simulink model "FormalArchitecture"  (R2022a)
settings: Solver=VariableStepAuto  StartTime=0.0  StopTime=10.0  RelTol=1e-3
settings Model: Creator=jdelolmo  LastModifiedBy=jdelolmo

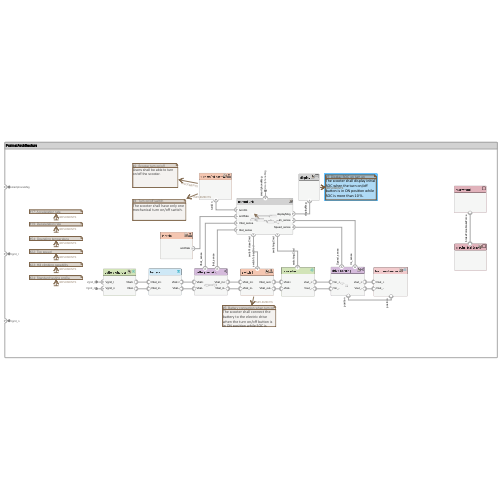
[thumbnail: Simulink's stored preview of the top-level diagram]
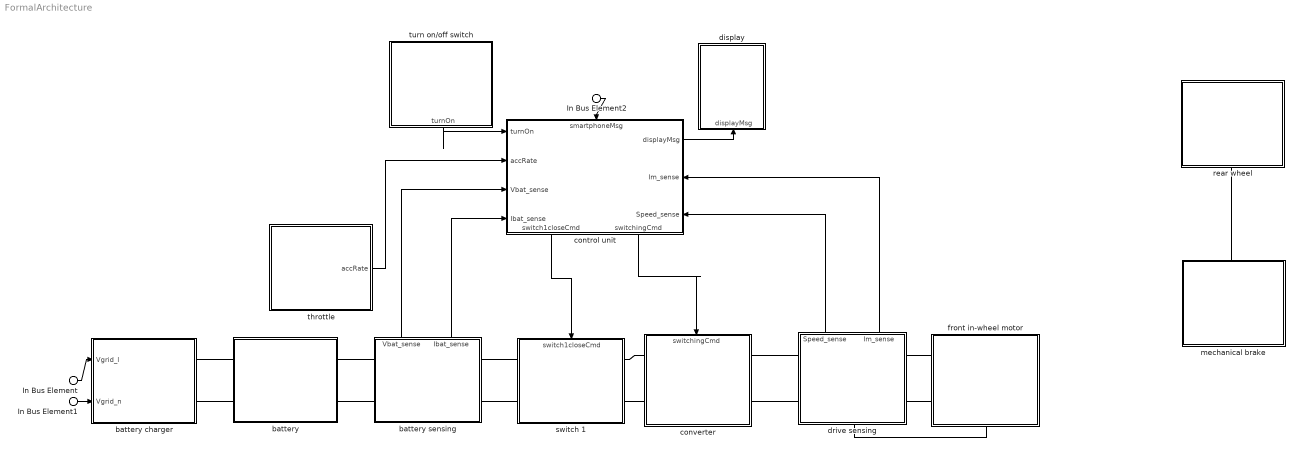
== system FormalArchitecture ==
  In Bus Element2 : Inport  PortName=smartphoneMsg
  In Bus Element : Inport  Port=2  PortName=Vgrid_l
  In Bus Element1 : Inport  Port=3  PortName=Vgrid_n
  battery : Subsystem
      settings: PortSchema="{\"entries\":[{\"content\":{\"headerSize\":26,\"margin\":15,\"minimumSpacing\":25,\"sides\":[{\"content\":{\"connectorIds\":[\"RConn1\",\"RConn2\"]},\"type\":\"ConnectorPlacement.EquallySpacedRectSide\",\"uuid\":\"ee500202-9322-4fb0-a7cb-dad4ec0e2ec3\"},{\"content\":{\"connectorIds\":[\"RConn3\",\"RConn4\"],\"side\":\"RIGHT\"},\"type\":\"ConnectorPlacement.EquallySpacedRectSide\",\"uuid\":\"837fb5dd-499e-46ad-8a25-662d532e1a52\"},{\"content\":{\"connectorIds\":[],\"side\":\"TOP\"},\"type\":\"ConnectorPlacement.EquallySpacedRectSide\",\"uuid\":\"1d32fa59-c030-426a-a0dc-2698c9a02a9b\"},{\"content\":{\"connectorIds\":[],\"side\":\"BOTTOM\"},\"type\":\"ConnectorPlacement.EquallySpacedRectSide\",\"uuid\":\"eb3de403-861e-4d45-8877-523b8cecc4fc\"}]},\"type\":\"ConnectorPlacement.EquallySpacedConnector\",\"uuid\":\"b24d61c9-c26d-4c33-81cf-af7207f0b73c\"}],\"packageUris\":[\"http://schema.mathworks.com/mf0/Connector/R2020b\"],\"version\":\"1.0\"}"
  battery charger : Subsystem
      settings: PortSchema="{\"entries\":[{\"content\":{\"headerSize\":26,\"margin\":15,\"minimumSpacing\":25,\"sides\":[{\"content\":{\"connectorIds\":[\"In1\",\"In2\"]},\"type\":\"ConnectorPlacement.EquallySpacedRectSide\",\"uuid\":\"77baa894-24de-420f-bb05-d29ca1eca7c3\"},{\"content\":{\"connectorIds\":[\"RConn1\",\"RConn2\"],\"side\":\"RIGHT\"},\"type\":\"ConnectorPlacement.EquallySpacedRectSide\",\"uuid\":\"fcd1216d-879c-477b-b249-00119a9fcd22\"},{\"content\":{\"connectorIds\":[],\"side\":\"TOP\"},\"type\":\"ConnectorPlacement.EquallySpacedRectSide\",\"uuid\":\"8485fad0-b9d7-4909-af21-eb521f98cd52\"}]},\"type\":\"ConnectorPlacement.EquallySpacedConnector\",\"uuid\":\"ff53bada-a376-4b82-92cc-106e9afccafe\"}],\"packageUris\":[\"http://schema.mathworks.com/mf0/Connector/R2020b\"],\"version\":\"1.0\"}"
  battery sensing : Subsystem
      settings: PortSchema="{\"entries\":[{\"content\":{\"headerSize\":26,\"margin\":15,\"minimumSpacing\":25,\"sides\":[{\"content\":{\"connectorIds\":[\"LConn1\",\"LConn2\"]},\"type\":\"ConnectorPlacement.EquallySpacedRectSide\",\"uuid\":\"77baa894-24de-420f-bb05-d29ca1eca7c3\"},{\"content\":{\"connectorIds\":[\"RConn1\",\"RConn2\"],\"side\":\"RIGHT\"},\"type\":\"ConnectorPlacement.EquallySpacedRectSide\",\"uuid\":\"fcd1216d-879c-477b-b249-00119a9fcd22\"},{\"content\":{\"connectorIds\":[\"Out2\",\"Out1\"],\"side\":\"TOP\"},\"type\":\"ConnectorPlacement.EquallySpacedRectSide\",\"uuid\":\"8485fad0-b9d7-4909-af21-eb521f98cd52\"},{\"content\":{\"connectorIds\":[],\"side\":\"BOTTOM\"},\"type\":\"ConnectorPlacement.EquallySpacedRectSide\",\"uuid\":\"41cb2969-f54e-4140-878a-5f5a3199a51a\"}]},\"type\":\"ConnectorPlacement.EquallySpacedConnector\",\"uuid\":\"ff53bada-a376-4b82-92cc-106e9afccafe\"}],\"packageUris\":[\"http://schema.mathworks.com/mf0/Connector/R2020b\"],\"version\":\"1.0\"}"
  control unit : Subsystem
      settings: PortSchema="{\"entries\":[{\"content\":{\"headerSize\":26,\"margin\":15,\"minimumSpacing\":25,\"sides\":[{\"content\":{\"connectorIds\":[\"In6\",\"In7\",\"In4\",\"In5\"]},\"type\":\"ConnectorPlacement.EquallySpacedRectSide\",\"uuid\":\"77baa894-24de-420f-bb05-d29ca1eca7c3\"},{\"content\":{\"connectorIds\":[\"Out1\",\"In2\",\"In3\"],\"side\":\"RIGHT\"},\"type\":\"ConnectorPlacement.EquallySpacedRectSide\",\"uuid\":\"fcd1216d-879c-477b-b249-00119a9fcd22\"},{\"content\":{\"connectorIds\":[\"In1\"],\"side\":\"TOP\"},\"type\":\"ConnectorPlacement.EquallySpacedRectSide\",\"uuid\":\"8485fad0-b9d7-4909-af21-eb521f98cd52\"},{\"content\":{\"connectorIds\":[\"Out3\",\"Out2\"],\"side\":\"BOTTOM\"},\"type\":\"ConnectorPlacement.EquallySpacedRectSide\",\"uuid\":\"7527fd4a-b56c-444b-9faf-560b8cff8cb7\"}]},\"type\":\"ConnectorPlacement.EquallySpacedConnector\",\"uuid\":\"ff53bada-a376-4b82-92cc-106e9afccafe\"}],\"packageUris\":[\"http://schema.mathworks.com/mf0/Connector/R2020b\"],\"version\":\"1.0\"}"
  converter : Subsystem
      settings: PortSchema="{\"entries\":[{\"content\":{\"headerSize\":26,\"margin\":15,\"minimumSpacing\":25,\"sides\":[{\"content\":{\"connectorIds\":[\"LConn1\",\"LConn2\"]},\"type\":\"ConnectorPlacement.EquallySpacedRectSide\",\"uuid\":\"77baa894-24de-420f-bb05-d29ca1eca7c3\"},{\"content\":{\"connectorIds\":[\"RConn1\",\"RConn2\"],\"side\":\"RIGHT\"},\"type\":\"ConnectorPlacement.EquallySpacedRectSide\",\"uuid\":\"fcd1216d-879c-477b-b249-00119a9fcd22\"},{\"content\":{\"connectorIds\":[\"In1\"],\"side\":\"TOP\"},\"type\":\"ConnectorPlacement.EquallySpacedRectSide\",\"uuid\":\"8485fad0-b9d7-4909-af21-eb521f98cd52\"}]},\"type\":\"ConnectorPlacement.EquallySpacedConnector\",\"uuid\":\"ff53bada-a376-4b82-92cc-106e9afccafe\"}],\"packageUris\":[\"http://schema.mathworks.com/mf0/Connector/R2020b\"],\"version\":\"1.0\"}"
  display : Subsystem
      settings: PortSchema="{\"entries\":[{\"content\":{\"headerSize\":26,\"margin\":15,\"minimumSpacing\":25,\"sides\":[{\"content\":{\"connectorIds\":[]},\"type\":\"ConnectorPlacement.EquallySpacedRectSide\",\"uuid\":\"77baa894-24de-420f-bb05-d29ca1eca7c3\"},{\"content\":{\"connectorIds\":[],\"side\":\"RIGHT\"},\"type\":\"ConnectorPlacement.EquallySpacedRectSide\",\"uuid\":\"fcd1216d-879c-477b-b249-00119a9fcd22\"},{\"content\":{\"connectorIds\":[],\"side\":\"TOP\"},\"type\":\"ConnectorPlacement.EquallySpacedRectSide\",\"uuid\":\"8485fad0-b9d7-4909-af21-eb521f98cd52\"},{\"content\":{\"connectorIds\":[\"In1\"],\"side\":\"BOTTOM\"},\"type\":\"ConnectorPlacement.EquallySpacedRectSide\",\"uuid\":\"2af0670b-3d52-4fa1-839f-7a09c90230ed\"}]},\"type\":\"ConnectorPlacement.EquallySpacedConnector\",\"uuid\":\"ff53bada-a376-4b82-92cc-106e9afccafe\"}],\"packageUris\":[\"http://schema.mathworks.com/mf0/Connector/R2020b\"],\"version\":\"1.0\"}"
  drive sensing : Subsystem
      settings: PortSchema="{\"entries\":[{\"content\":{\"headerSize\":26,\"margin\":15,\"minimumSpacing\":25,\"sides\":[{\"content\":{\"connectorIds\":[\"LConn1\",\"LConn2\"]},\"type\":\"ConnectorPlacement.EquallySpacedRectSide\",\"uuid\":\"77baa894-24de-420f-bb05-d29ca1eca7c3\"},{\"content\":{\"connectorIds\":[\"RConn2\",\"RConn3\"],\"side\":\"RIGHT\"},\"type\":\"ConnectorPlacement.EquallySpacedRectSide\",\"uuid\":\"fcd1216d-879c-477b-b249-00119a9fcd22\"},{\"content\":{\"connectorIds\":[\"Out1\",\"Out2\"],\"side\":\"TOP\"},\"type\":\"ConnectorPlacement.EquallySpacedRectSide\",\"uuid\":\"8485fad0-b9d7-4909-af21-eb521f98cd52\"},{\"content\":{\"connectorIds\":[\"RConn1\"],\"side\":\"BOTTOM\"},\"type\":\"ConnectorPlacement.EquallySpacedRectSide\",\"uuid\":\"d4cb5d60-5908-4c53-8bc7-b25c3bd545d1\"}]},\"type\":\"ConnectorPlacement.EquallySpacedConnector\",\"uuid\":\"ff53bada-a376-4b82-92cc-106e9afccafe\"}],\"packageUris\":[\"http://schema.mathworks.com/mf0/Connector/R2020b\"],\"version\":\"1.0\"}"
  front in-wheel motor : Subsystem
      settings: PortSchema="{\"entries\":[{\"content\":{\"headerSize\":26,\"margin\":15,\"minimumSpacing\":25,\"sides\":[{\"content\":{\"connectorIds\":[\"LConn1\",\"LConn2\"]},\"type\":\"ConnectorPlacement.EquallySpacedRectSide\",\"uuid\":\"77baa894-24de-420f-bb05-d29ca1eca7c3\"},{\"content\":{\"connectorIds\":[],\"side\":\"RIGHT\"},\"type\":\"ConnectorPlacement.EquallySpacedRectSide\",\"uuid\":\"fcd1216d-879c-477b-b249-00119a9fcd22\"},{\"content\":{\"connectorIds\":[],\"side\":\"TOP\"},\"type\":\"ConnectorPlacement.EquallySpacedRectSide\",\"uuid\":\"8485fad0-b9d7-4909-af21-eb521f98cd52\"},{\"content\":{\"connectorIds\":[\"RConn1\"],\"side\":\"BOTTOM\"},\"type\":\"ConnectorPlacement.EquallySpacedRectSide\",\"uuid\":\"b1cf9e87-5a5a-4f73-9ce1-9d94c90c7687\"}]},\"type\":\"ConnectorPlacement.EquallySpacedConnector\",\"uuid\":\"ff53bada-a376-4b82-92cc-106e9afccafe\"}],\"packageUris\":[\"http://schema.mathworks.com/mf0/Connector/R2020b\"],\"version\":\"1.0\"}"
  mechanical brake : Subsystem
      settings: PortSchema="{\"entries\":[{\"content\":{\"headerSize\":26,\"margin\":15,\"minimumSpacing\":25,\"sides\":[{\"content\":{\"connectorIds\":[]},\"type\":\"ConnectorPlacement.EquallySpacedRectSide\",\"uuid\":\"77baa894-24de-420f-bb05-d29ca1eca7c3\"},{\"content\":{\"connectorIds\":[],\"side\":\"RIGHT\"},\"type\":\"ConnectorPlacement.EquallySpacedRectSide\",\"uuid\":\"fcd1216d-879c-477b-b249-00119a9fcd22\"},{\"content\":{\"connectorIds\":[\"LConn1\"],\"side\":\"TOP\"},\"type\":\"ConnectorPlacement.EquallySpacedRectSide\",\"uuid\":\"8485fad0-b9d7-4909-af21-eb521f98cd52\"}]},\"type\":\"ConnectorPlacement.EquallySpacedConnector\",\"uuid\":\"ff53bada-a376-4b82-92cc-106e9afccafe\"}],\"packageUris\":[\"http://schema.mathworks.com/mf0/Connector/R2020b\"],\"version\":\"1.0\"}"
  rear wheel : Subsystem
      settings: PortSchema="{\"entries\":[{\"content\":{\"headerSize\":26,\"margin\":15,\"minimumSpacing\":25,\"sides\":[{\"content\":{\"connectorIds\":[]},\"type\":\"ConnectorPlacement.EquallySpacedRectSide\",\"uuid\":\"77baa894-24de-420f-bb05-d29ca1eca7c3\"},{\"content\":{\"connectorIds\":[],\"side\":\"RIGHT\"},\"type\":\"ConnectorPlacement.EquallySpacedRectSide\",\"uuid\":\"fcd1216d-879c-477b-b249-00119a9fcd22\"},{\"content\":{\"connectorIds\":[],\"side\":\"TOP\"},\"type\":\"ConnectorPlacement.EquallySpacedRectSide\",\"uuid\":\"8485fad0-b9d7-4909-af21-eb521f98cd52\"},{\"content\":{\"connectorIds\":[\"RConn1\"],\"side\":\"BOTTOM\"},\"type\":\"ConnectorPlacement.EquallySpacedRectSide\",\"uuid\":\"21d572fb-02a4-48d3-884f-e95f709af539\"}]},\"type\":\"ConnectorPlacement.EquallySpacedConnector\",\"uuid\":\"ff53bada-a376-4b82-92cc-106e9afccafe\"}],\"packageUris\":[\"http://schema.mathworks.com/mf0/Connector/R2020b\"],\"version\":\"1.0\"}"
  switch 1 : Subsystem
      settings: PortSchema="{\"entries\":[{\"content\":{\"headerSize\":26,\"margin\":15,\"minimumSpacing\":25,\"sides\":[{\"content\":{\"connectorIds\":[\"LConn1\",\"LConn2\"]},\"type\":\"ConnectorPlacement.EquallySpacedRectSide\",\"uuid\":\"77baa894-24de-420f-bb05-d29ca1eca7c3\"},{\"content\":{\"connectorIds\":[\"RConn1\",\"RConn2\"],\"side\":\"RIGHT\"},\"type\":\"ConnectorPlacement.EquallySpacedRectSide\",\"uuid\":\"fcd1216d-879c-477b-b249-00119a9fcd22\"},{\"content\":{\"connectorIds\":[\"In1\"],\"side\":\"TOP\"},\"type\":\"ConnectorPlacement.EquallySpacedRectSide\",\"uuid\":\"8485fad0-b9d7-4909-af21-eb521f98cd52\"}]},\"type\":\"ConnectorPlacement.EquallySpacedConnector\",\"uuid\":\"ff53bada-a376-4b82-92cc-106e9afccafe\"}],\"packageUris\":[\"http://schema.mathworks.com/mf0/Connector/R2020b\"],\"version\":\"1.0\"}"
  throttle : Subsystem
      settings: PortSchema="{\"entries\":[{\"content\":{\"headerSize\":26,\"margin\":15,\"minimumSpacing\":25,\"sides\":[{\"content\":{\"connectorIds\":[]},\"type\":\"ConnectorPlacement.EquallySpacedRectSide\",\"uuid\":\"77baa894-24de-420f-bb05-d29ca1eca7c3\"},{\"content\":{\"connectorIds\":[\"Out1\"],\"side\":\"RIGHT\"},\"type\":\"ConnectorPlacement.EquallySpacedRectSide\",\"uuid\":\"fcd1216d-879c-477b-b249-00119a9fcd22\"},{\"content\":{\"connectorIds\":[],\"side\":\"TOP\"},\"type\":\"ConnectorPlacement.EquallySpacedRectSide\",\"uuid\":\"8485fad0-b9d7-4909-af21-eb521f98cd52\"}]},\"type\":\"ConnectorPlacement.EquallySpacedConnector\",\"uuid\":\"ff53bada-a376-4b82-92cc-106e9afccafe\"}],\"packageUris\":[\"http://schema.mathworks.com/mf0/Connector/R2020b\"],\"version\":\"1.0\"}"
  turn on/off switch : Subsystem
      settings: PortSchema="{\"entries\":[{\"content\":{\"headerSize\":26,\"margin\":15,\"minimumSpacing\":25,\"sides\":[{\"content\":{\"connectorIds\":[]},\"type\":\"ConnectorPlacement.EquallySpacedRectSide\",\"uuid\":\"77baa894-24de-420f-bb05-d29ca1eca7c3\"},{\"content\":{\"connectorIds\":[],\"side\":\"RIGHT\"},\"type\":\"ConnectorPlacement.EquallySpacedRectSide\",\"uuid\":\"fcd1216d-879c-477b-b249-00119a9fcd22\"},{\"content\":{\"connectorIds\":[],\"side\":\"TOP\"},\"type\":\"ConnectorPlacement.EquallySpacedRectSide\",\"uuid\":\"8485fad0-b9d7-4909-af21-eb521f98cd52\"},{\"content\":{\"connectorIds\":[\"Out1\"],\"side\":\"BOTTOM\"},\"type\":\"ConnectorPlacement.EquallySpacedRectSide\",\"uuid\":\"39085245-15cc-4ad1-9a37-6dd6a1d598c8\"}]},\"type\":\"ConnectorPlacement.EquallySpacedConnector\",\"uuid\":\"ff53bada-a376-4b82-92cc-106e9afccafe\"}],\"packageUris\":[\"http://schema.mathworks.com/mf0/Connector/R2020b\"],\"version\":\"1.0\"}"
  wires:
  turn on/off switch/1(turnOn) -> control unit/6(turnOn)
  control unit/3(switch1closeCmd) -> switch 1/1(switch1closeCmd)
  control unit/1(displayMsg) -> display/1(displayMsg)
  throttle/1(accRate) -> control unit/7(accRate)
  battery sensing/2(Vbat_sense) -> control unit/4(Vbat_sense)
  battery sensing/1(Ibat_sense) -> control unit/5(Ibat_sense)
  drive sensing/2(Im_sense) -> control unit/2(Im_sense)
  drive sensing/1(Speed_sense) -> control unit/3(Speed_sense)
  In Bus Element/1 -> battery charger/1(Vgrid_l)
  In Bus Element1/1 -> battery charger/2(Vgrid_n)
  In Bus Element2/1 -> control unit/1(smartphoneMsg)
  control unit/2(switchingCmd) -> converter/1(switchingCmd)
  connections:
  converter/LConn1 -- switch 1/RConn1
  converter/LConn2 -- switch 1/RConn2
  switch 1/LConn1 -- battery sensing/RConn1
  switch 1/LConn2 -- battery sensing/RConn2
  converter/RConn1 -- drive sensing/LConn1
  converter/RConn2 -- drive sensing/LConn2
  front in-wheel motor/LConn1 -- drive sensing/RConn2
  front in-wheel motor/LConn2 -- drive sensing/RConn3
  drive sensing/RConn1 -- front in-wheel motor/RConn1
  mechanical brake/LConn1 -- rear wheel/RConn1
  battery sensing/LConn1 -- battery/RConn3
  battery sensing/LConn2 -- battery/RConn4
  battery charger/RConn1 -- battery/RConn1
  battery charger/RConn2 -- battery/RConn2

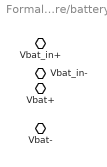
== system FormalArchitecture/battery ==
  Vbat_in+ : PMIOPort  Side=Right
  Vbat_in- : PMIOPort  Port=2  Side=Right
  Vbat+ : PMIOPort  Port=3  Side=Right
  Vbat- : PMIOPort  Port=4  Side=Right

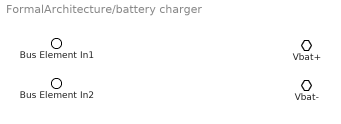
== system FormalArchitecture/battery charger ==
  Bus Element In1 : Inport  PortName=Vgrid_l
  Bus Element In2 : Inport  Port=2  PortName=Vgrid_n
  Vbat+ : PMIOPort  Side=Right
  Vbat- : PMIOPort  Port=2  Side=Right

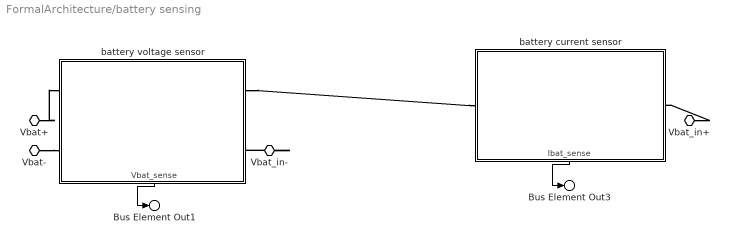
== system FormalArchitecture/battery sensing ==
  battery current sensor : Subsystem
      settings: PortSchema="{\"entries\":[{\"content\":{\"headerSize\":26,\"margin\":15,\"minimumSpacing\":25,\"sides\":[{\"content\":{\"connectorIds\":[\"LConn1\"]},\"type\":\"ConnectorPlacement.EquallySpacedRectSide\",\"uuid\":\"77baa894-24de-420f-bb05-d29ca1eca7c3\"},{\"content\":{\"connectorIds\":[\"RConn1\"],\"side\":\"RIGHT\"},\"type\":\"ConnectorPlacement.EquallySpacedRectSide\",\"uuid\":\"fcd1216d-879c-477b-b249-00119a9fcd22\"},{\"content\":{\"connectorIds\":[],\"side\":\"TOP\"},\"type\":\"ConnectorPlacement.EquallySpacedRectSide\",\"uuid\":\"8485fad0-b9d7-4909-af21-eb521f98cd52\"},{\"content\":{\"connectorIds\":[\"Out1\"],\"side\":\"BOTTOM\"},\"type\":\"ConnectorPlacement.EquallySpacedRectSide\",\"uuid\":\"b087b9fb-29ea-43eb-a167-2ce7aba8e49e\"}]},\"type\":\"ConnectorPlacement.EquallySpacedConnector\",\"uuid\":\"ff53bada-a376-4b82-92cc-106e9afccafe\"}],\"packageUris\":[\"http://schema.mathworks.com/mf0/Connector/R2020b\"],\"version\":\"1.0\"}"
  battery voltage sensor : Subsystem
      settings: PortSchema="{\"entries\":[{\"content\":{\"headerSize\":26,\"margin\":15,\"minimumSpacing\":25,\"sides\":[{\"content\":{\"connectorIds\":[\"LConn1\",\"LConn2\"]},\"type\":\"ConnectorPlacement.EquallySpacedRectSide\",\"uuid\":\"77baa894-24de-420f-bb05-d29ca1eca7c3\"},{\"content\":{\"connectorIds\":[\"RConn1\",\"RConn2\"],\"side\":\"RIGHT\"},\"type\":\"ConnectorPlacement.EquallySpacedRectSide\",\"uuid\":\"fcd1216d-879c-477b-b249-00119a9fcd22\"},{\"content\":{\"connectorIds\":[],\"side\":\"TOP\"},\"type\":\"ConnectorPlacement.EquallySpacedRectSide\",\"uuid\":\"8485fad0-b9d7-4909-af21-eb521f98cd52\"},{\"content\":{\"connectorIds\":[\"Out1\"],\"side\":\"BOTTOM\"},\"type\":\"ConnectorPlacement.EquallySpacedRectSide\",\"uuid\":\"04039fcf-9b1b-4283-ba0c-bcd076f35720\"}]},\"type\":\"ConnectorPlacement.EquallySpacedConnector\",\"uuid\":\"ff53bada-a376-4b82-92cc-106e9afccafe\"}],\"packageUris\":[\"http://schema.mathworks.com/mf0/Connector/R2020b\"],\"version\":\"1.0\"}"
  Vbat+ : PMIOPort  Side=Left
  Vbat- : PMIOPort  Port=2  Side=Left
  Vbat_in+ : PMIOPort  Port=3  Side=Right
  Vbat_in- : PMIOPort  Port=4  Side=Right
  Bus Element Out3 : Outport  PortName=Ibat_sense
  Bus Element Out1 : Outport  Port=2  PortName=Vbat_sense
  wires:
  battery voltage sensor/1(Vbat_sense) -> Bus Element Out1/1
  battery current sensor/1(Ibat_sense) -> Bus Element Out3/1
  connections:
  Vbat+/RConn1 -- battery voltage sensor/LConn1
  Vbat-/RConn1 -- battery voltage sensor/LConn2
  Vbat_in-/RConn1 -- battery voltage sensor/RConn2
  battery voltage sensor/RConn1 -- battery current sensor/LConn1
  Vbat_in+/RConn1 -- battery current sensor/RConn1

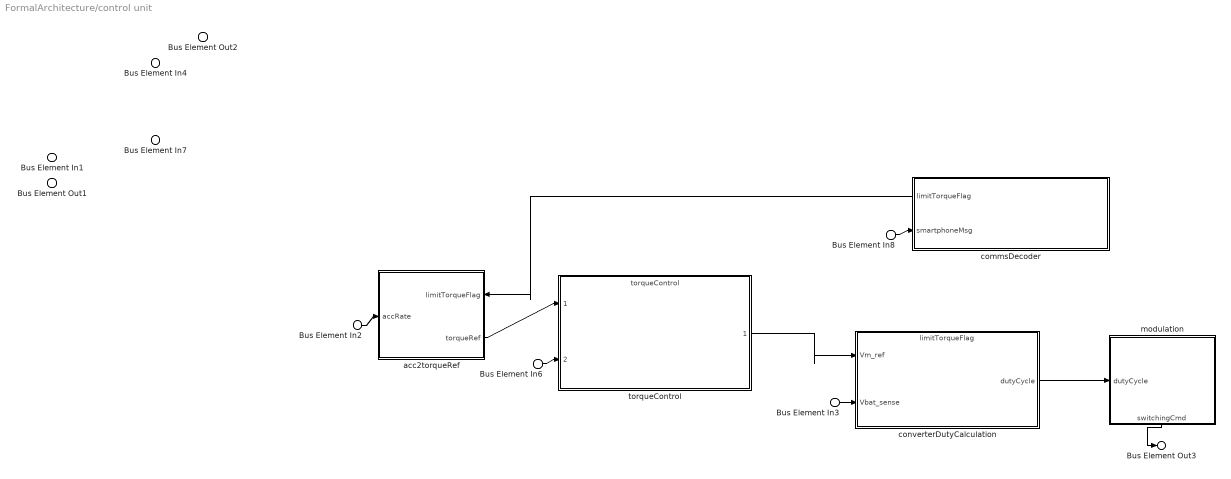
== system FormalArchitecture/control unit ==
  Bus Element In8 : Inport  PortName=smartphoneMsg
  Bus Element In6 : Inport  Port=2  PortName=Im_sense
  Bus Element In7 : Inport  Port=3  PortName=Speed_sense
  Bus Element In3 : Inport  Port=4  PortName=Vbat_sense
  Bus Element In4 : Inport  Port=5  PortName=Ibat_sense
  Bus Element In1 : Inport  Port=6  PortName=turnOn
  Bus Element In2 : Inport  Port=7  PortName=accRate
  acc2torqueRef : Subsystem
      settings: PortSchema="{\"entries\":[{\"content\":{\"headerSize\":26,\"margin\":15,\"minimumSpacing\":25,\"sides\":[{\"content\":{\"connectorIds\":[\"In2\"]},\"type\":\"ConnectorPlacement.EquallySpacedRectSide\",\"uuid\":\"c417387f-860e-41c8-9911-3c50efe17f0f\"},{\"content\":{\"connectorIds\":[\"In1\",\"Out1\"],\"side\":\"RIGHT\"},\"type\":\"ConnectorPlacement.EquallySpacedRectSide\",\"uuid\":\"91196307-25cf-4e7f-8b62-2e4af4ce1698\"},{\"content\":{\"connectorIds\":[],\"side\":\"TOP\"},\"type\":\"ConnectorPlacement.EquallySpacedRectSide\",\"uuid\":\"ebdf9ca0-c77b-4c6e-90f0-033a6299dca5\"},{\"content\":{\"connectorIds\":[],\"side\":\"BOTTOM\"},\"type\":\"ConnectorPlacement.EquallySpacedRectSide\",\"uuid\":\"1b3f30f3-99be-4f51-9ca5-a3fb99d93d5a\"}]},\"type\":\"ConnectorPlacement.EquallySpacedConnector\",\"uuid\":\"f2a2883c-4823-4841-afea-79946d01ae49\"}],\"packageUris\":[\"http://schema.mathworks.com/mf0/Connector/R2020b\"],\"version\":\"1.0\"}"
  commsDecoder : Subsystem
      settings: PortSchema="{\"entries\":[{\"content\":{\"headerSize\":26,\"margin\":15,\"minimumSpacing\":25,\"sides\":[{\"content\":{\"connectorIds\":[\"Out1\",\"In1\"]},\"type\":\"ConnectorPlacement.EquallySpacedRectSide\",\"uuid\":\"77baa894-24de-420f-bb05-d29ca1eca7c3\"},{\"content\":{\"connectorIds\":[],\"side\":\"RIGHT\"},\"type\":\"ConnectorPlacement.EquallySpacedRectSide\",\"uuid\":\"fcd1216d-879c-477b-b249-00119a9fcd22\"},{\"content\":{\"connectorIds\":[],\"side\":\"TOP\"},\"type\":\"ConnectorPlacement.EquallySpacedRectSide\",\"uuid\":\"8485fad0-b9d7-4909-af21-eb521f98cd52\"}]},\"type\":\"ConnectorPlacement.EquallySpacedConnector\",\"uuid\":\"ff53bada-a376-4b82-92cc-106e9afccafe\"}],\"packageUris\":[\"http://schema.mathworks.com/mf0/Connector/R2020b\"],\"version\":\"1.0\"}"
  converterDutyCalculation : Subsystem
      settings: PortSchema="{\"entries\":[{\"content\":{\"headerSize\":26,\"margin\":15,\"minimumSpacing\":25,\"sides\":[{\"content\":{\"connectorIds\":[\"In1\",\"In2\"]},\"type\":\"ConnectorPlacement.EquallySpacedRectSide\",\"uuid\":\"c417387f-860e-41c8-9911-3c50efe17f0f\"},{\"content\":{\"connectorIds\":[\"Out1\"],\"side\":\"RIGHT\"},\"type\":\"ConnectorPlacement.EquallySpacedRectSide\",\"uuid\":\"91196307-25cf-4e7f-8b62-2e4af4ce1698\"},{\"content\":{\"connectorIds\":[\"In3\"],\"side\":\"TOP\"},\"type\":\"ConnectorPlacement.EquallySpacedRectSide\",\"uuid\":\"ebdf9ca0-c77b-4c6e-90f0-033a6299dca5\"},{\"content\":{\"connectorIds\":[],\"side\":\"BOTTOM\"},\"type\":\"ConnectorPlacement.EquallySpacedRectSide\",\"uuid\":\"1b3f30f3-99be-4f51-9ca5-a3fb99d93d5a\"}]},\"type\":\"ConnectorPlacement.EquallySpacedConnector\",\"uuid\":\"f2a2883c-4823-4841-afea-79946d01ae49\"}],\"packageUris\":[\"http://schema.mathworks.com/mf0/Connector/R2020b\"],\"version\":\"1.0\"}"
  modulation : Subsystem
      settings: PortSchema="{\"entries\":[{\"content\":{\"headerSize\":26,\"margin\":15,\"minimumSpacing\":25,\"sides\":[{\"content\":{\"connectorIds\":[\"In1\"]},\"type\":\"ConnectorPlacement.EquallySpacedRectSide\",\"uuid\":\"c417387f-860e-41c8-9911-3c50efe17f0f\"},{\"content\":{\"connectorIds\":[],\"side\":\"RIGHT\"},\"type\":\"ConnectorPlacement.EquallySpacedRectSide\",\"uuid\":\"91196307-25cf-4e7f-8b62-2e4af4ce1698\"},{\"content\":{\"connectorIds\":[],\"side\":\"TOP\"},\"type\":\"ConnectorPlacement.EquallySpacedRectSide\",\"uuid\":\"ebdf9ca0-c77b-4c6e-90f0-033a6299dca5\"},{\"content\":{\"connectorIds\":[\"Out1\"],\"side\":\"BOTTOM\"},\"type\":\"ConnectorPlacement.EquallySpacedRectSide\",\"uuid\":\"339ed08e-3e32-467a-8159-dcf3620fc7b7\"}]},\"type\":\"ConnectorPlacement.EquallySpacedConnector\",\"uuid\":\"f2a2883c-4823-4841-afea-79946d01ae49\"}],\"packageUris\":[\"http://schema.mathworks.com/mf0/Connector/R2020b\"],\"version\":\"1.0\"}"
  torqueControl : ModelReference  ModelNameDialog=torqueControl  SimulationMode=Normal  ModelReferenceVersion=1.4
      settings: PortSchema="{\"entries\":[{\"content\":{\"headerSize\":38,\"margin\":15,\"minimumSpacing\":25,\"sides\":[{\"content\":{\"connectorIds\":[\"In1\",\"In2\"]},\"type\":\"ConnectorPlacement.EquallySpacedRectSide\",\"uuid\":\"c417387f-860e-41c8-9911-3c50efe17f0f\"},{\"content\":{\"connectorIds\":[\"Out1\"],\"side\":\"RIGHT\"},\"type\":\"ConnectorPlacement.EquallySpacedRectSide\",\"uuid\":\"91196307-25cf-4e7f-8b62-2e4af4ce1698\"},{\"content\":{\"connectorIds\":[],\"side\":\"TOP\"},\"type\":\"ConnectorPlacement.EquallySpacedRectSide\",\"uuid\":\"ebdf9ca0-c77b-4c6e-90f0-033a6299dca5\"},{\"content\":{\"connectorIds\":[],\"side\":\"BOTTOM\"},\"type\":\"ConnectorPlacement.EquallySpacedRectSide\",\"uuid\":\"1b3f30f3-99be-4f51-9ca5-a3fb99d93d5a\"}]},\"type\":\"ConnectorPlacement.EquallySpacedConnector\",\"uuid\":\"f2a2883c-4823-4841-afea-79946d01ae49\"}],\"packageUris\":[\"http://schema.mathworks.com/mf0/Connector/R2020b\"],\"version\":\"1.0\"}"
  Bus Element Out2 : Outport  PortName=displayMsg
  Bus Element Out3 : Outport  Port=2  PortName=switchingCmd
  Bus Element Out1 : Outport  Port=3  PortName=switch1closeCmd
  wires:
  Bus Element In8/1 -> commsDecoder/1(smartphoneMsg)
  Bus Element In2/1 -> acc2torqueRef/2(accRate)
  Bus Element In3/1 -> converterDutyCalculation/2(Vbat_sense)
  converterDutyCalculation/1(dutyCycle) -> modulation/1(dutyCycle)
  modulation/1(switchingCmd) -> Bus Element Out3/1
  commsDecoder/1(limitTorqueFlag) -> acc2torqueRef/1(limitTorqueFlag)
  Bus Element In6/1 -> torqueControl/2
  acc2torqueRef/1(torqueRef) -> torqueControl/1
  torqueControl/1 -> converterDutyCalculation/1(Vm_ref)

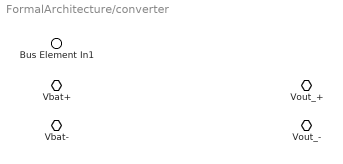
== system FormalArchitecture/converter ==
  Bus Element In1 : Inport  PortName=switchingCmd
  Vbat+ : PMIOPort  Side=Left
  Vbat- : PMIOPort  Port=2  Side=Left
  Vout_+ : PMIOPort  Port=3  Side=Right
  Vout_- : PMIOPort  Port=4  Side=Right

== system FormalArchitecture/display ==
  Bus Element In1 : Inport  PortName=displayMsg

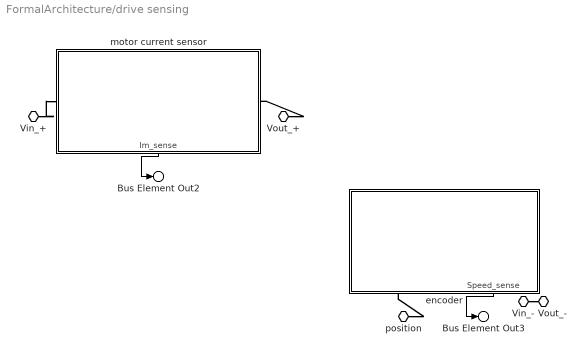
== system FormalArchitecture/drive sensing ==
  encoder : Subsystem
      settings: PortSchema="{\"entries\":[{\"content\":{\"headerSize\":26,\"margin\":15,\"minimumSpacing\":25,\"sides\":[{\"content\":{\"connectorIds\":[]},\"type\":\"ConnectorPlacement.EquallySpacedRectSide\",\"uuid\":\"77baa894-24de-420f-bb05-d29ca1eca7c3\"},{\"content\":{\"connectorIds\":[],\"side\":\"RIGHT\"},\"type\":\"ConnectorPlacement.EquallySpacedRectSide\",\"uuid\":\"fcd1216d-879c-477b-b249-00119a9fcd22\"},{\"content\":{\"connectorIds\":[],\"side\":\"TOP\"},\"type\":\"ConnectorPlacement.EquallySpacedRectSide\",\"uuid\":\"8485fad0-b9d7-4909-af21-eb521f98cd52\"},{\"content\":{\"connectorIds\":[\"RConn1\",\"Out1\"],\"side\":\"BOTTOM\"},\"type\":\"ConnectorPlacement.EquallySpacedRectSide\",\"uuid\":\"36307a6f-387a-4d32-ae7b-453251c763ef\"}]},\"type\":\"ConnectorPlacement.EquallySpacedConnector\",\"uuid\":\"ff53bada-a376-4b82-92cc-106e9afccafe\"}],\"packageUris\":[\"http://schema.mathworks.com/mf0/Connector/R2020b\"],\"version\":\"1.0\"}"
  motor current sensor : Subsystem
      settings: PortSchema="{\"entries\":[{\"content\":{\"headerSize\":26,\"margin\":15,\"minimumSpacing\":25,\"sides\":[{\"content\":{\"connectorIds\":[\"LConn1\"]},\"type\":\"ConnectorPlacement.EquallySpacedRectSide\",\"uuid\":\"77baa894-24de-420f-bb05-d29ca1eca7c3\"},{\"content\":{\"connectorIds\":[\"RConn1\"],\"side\":\"RIGHT\"},\"type\":\"ConnectorPlacement.EquallySpacedRectSide\",\"uuid\":\"fcd1216d-879c-477b-b249-00119a9fcd22\"},{\"content\":{\"connectorIds\":[],\"side\":\"TOP\"},\"type\":\"ConnectorPlacement.EquallySpacedRectSide\",\"uuid\":\"8485fad0-b9d7-4909-af21-eb521f98cd52\"},{\"content\":{\"connectorIds\":[\"Out1\"],\"side\":\"BOTTOM\"},\"type\":\"ConnectorPlacement.EquallySpacedRectSide\",\"uuid\":\"936848f8-b142-4c68-8d83-22c4dc88dd78\"}]},\"type\":\"ConnectorPlacement.EquallySpacedConnector\",\"uuid\":\"ff53bada-a376-4b82-92cc-106e9afccafe\"}],\"packageUris\":[\"http://schema.mathworks.com/mf0/Connector/R2020b\"],\"version\":\"1.0\"}"
  Vin_+ : PMIOPort  Side=Left
  Vin_- : PMIOPort  Port=2  Side=Left
  position : PMIOPort  Port=3  Side=Right
  Vout_+ : PMIOPort  Port=4  Side=Right
  Vout_- : PMIOPort  Port=5  Side=Right
  Bus Element Out3 : Outport  PortName=Speed_sense
  Bus Element Out2 : Outport  Port=2  PortName=Im_sense
  wires:
  encoder/1(Speed_sense) -> Bus Element Out3/1
  motor current sensor/1(Im_sense) -> Bus Element Out2/1
  connections:
  Vin_+/RConn1 -- motor current sensor/LConn1
  Vout_+/RConn1 -- motor current sensor/RConn1
  position/RConn1 -- encoder/RConn1
  Vin_-/RConn1 -- Vout_-/RConn1

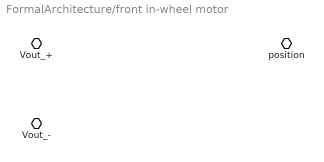
== system FormalArchitecture/front in-wheel motor ==
  Vout_+ : PMIOPort  Side=Left
  Vout_- : PMIOPort  Port=2  Side=Left
  position : PMIOPort  Port=3  Side=Right

== system FormalArchitecture/mechanical brake ==
  brakeForce : PMIOPort  Side=Left

== system FormalArchitecture/rear wheel ==
  brakeForce : PMIOPort  Side=Right

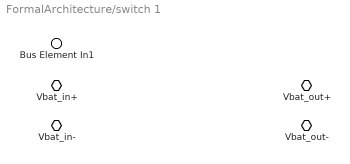
== system FormalArchitecture/switch 1 ==
  Bus Element In1 : Inport  PortName=switch1closeCmd
  Vbat_in+ : PMIOPort  Side=Left
  Vbat_in- : PMIOPort  Port=2  Side=Left
  Vbat_out+ : PMIOPort  Port=3  Side=Right
  Vbat_out- : PMIOPort  Port=4  Side=Right

== system FormalArchitecture/throttle ==
  Bus Element Out1 : Outport  PortName=accRate

== system FormalArchitecture/turn on//off switch ==
  Bus Element Out1 : Outport  PortName=turnOn

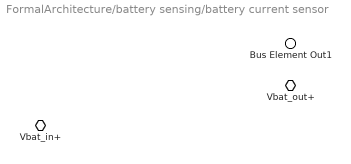
== system FormalArchitecture/battery sensing/battery current sensor ==
  Vbat_in+ : PMIOPort  Side=Left
  Vbat_out+ : PMIOPort  Port=2  Side=Right
  Bus Element Out1 : Outport  PortName=Ibat_sense

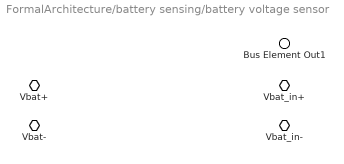
== system FormalArchitecture/battery sensing/battery voltage sensor ==
  Vbat+ : PMIOPort  Side=Left
  Vbat- : PMIOPort  Port=2  Side=Left
  Vbat_in+ : PMIOPort  Port=3  Side=Right
  Vbat_in- : PMIOPort  Port=4  Side=Right
  Bus Element Out1 : Outport  PortName=Vbat_sense

== system FormalArchitecture/control unit/acc2torqueRef ==
  Bus Element In2 : Inport  PortName=limitTorqueFlag
  Bus Element In1 : Inport  Port=2  PortName=accRate
  Bus Element Out1 : Outport  PortName=torqueRef

== system FormalArchitecture/control unit/commsDecoder ==
  Bus Element In1 : Inport  PortName=smartphoneMsg
  Bus Element Out1 : Outport  PortName=limitTorqueFlag

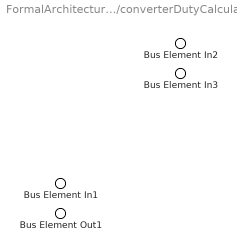
== system FormalArchitecture/control unit/converterDutyCalculation ==
  Bus Element In3 : Inport  PortName=Vm_ref
  Bus Element In2 : Inport  Port=2  PortName=Vbat_sense
  Bus Element In1 : Inport  Port=3  PortName=limitTorqueFlag
  Bus Element Out1 : Outport  PortName=dutyCycle

== system FormalArchitecture/control unit/modulation ==
  Bus Element In1 : Inport  PortName=dutyCycle
  Bus Element Out1 : Outport  PortName=switchingCmd

== system FormalArchitecture/drive sensing/encoder ==
  position : PMIOPort  Side=Right
  Bus Element Out1 : Outport  PortName=Speed_sense

== system FormalArchitecture/drive sensing/motor current sensor ==
  Vin_+ : PMIOPort  Side=Left
  Vout_- : PMIOPort  Port=2  Side=Right
  Bus Element Out1 : Outport  PortName=Im_sense
